simulink model "inverted_pendulum"  (Simulink 6.0)
settings: Solver=ode45  StartTime=0.0  StopTime=10.0  RelTol=1e-3
values from neighbouring files (symbols this model uses):
  B = [0;-1;0;1]    [Invertedpendulum.m]    (also in Untitled.m = [-1;0;2])
  C = eye(4)    [Invertedpendulum.m]    (also in Untitled.m = [0 1 0;0 0 1])
  C1 = C    [Invertedpendulum.m]
  C2 = C    [Invertedpendulum.m]
  C3 = C    [Invertedpendulum.m]
  C4 = C    [Invertedpendulum.m]
  E = [1;1;1;1]    [Invertedpendulum.m]    (also in Untitled.m = [1;0;1])
  F = diag(v)    [Invertedpendulum.m]    (also in Untitled.m = A1-K1'*C)
  F1 = T1*A-k11*C1    [Invertedpendulum.m]
  F3 = T3*A-k31*C3    [Invertedpendulum.m]
  F4 = T4*A-k41*C4    [Invertedpendulum.m]
  H = E*(inv((C*E)'*(C*E)))*(C*E)'    [Invertedpendulum.m]    (also in Untitled.m = E*inv((C*E)'*(C*E))*(C*E)')
  H1 = zeros(4,4)    [Invertedpendulum.m]
  H2 = zeros(4,4)    [Invertedpendulum.m]
  H3 = zeros(4,4)    [Invertedpendulum.m]
  H4 = zeros(4,4)    [Invertedpendulum.m]
  k = k1+k2    [Invertedpendulum.m]
  K1 = k11+k12    [Invertedpendulum.m]    (also in Untitled.m = place(A',C',[-2,-10,-5])')
  K2 = k21+k22    [Invertedpendulum.m]
  K3 = k31+k32    [Invertedpendulum.m]
  K4 = k41+k42    [Invertedpendulum.m]
  T = eye(4)-H*C    [Invertedpendulum.m]    (also in Untitled.m = eye(3)-H*C)
  T1 = eye(4)-H1*C1    [Invertedpendulum.m]
  T2 = eye(4)-H2*C2    [Invertedpendulum.m]
  T3 = eye(4)-H3*C3    [Invertedpendulum.m]
  T4 = eye(4)-H4*C4    [Invertedpendulum.m]
settings Model: LastModifiedBy=fel722

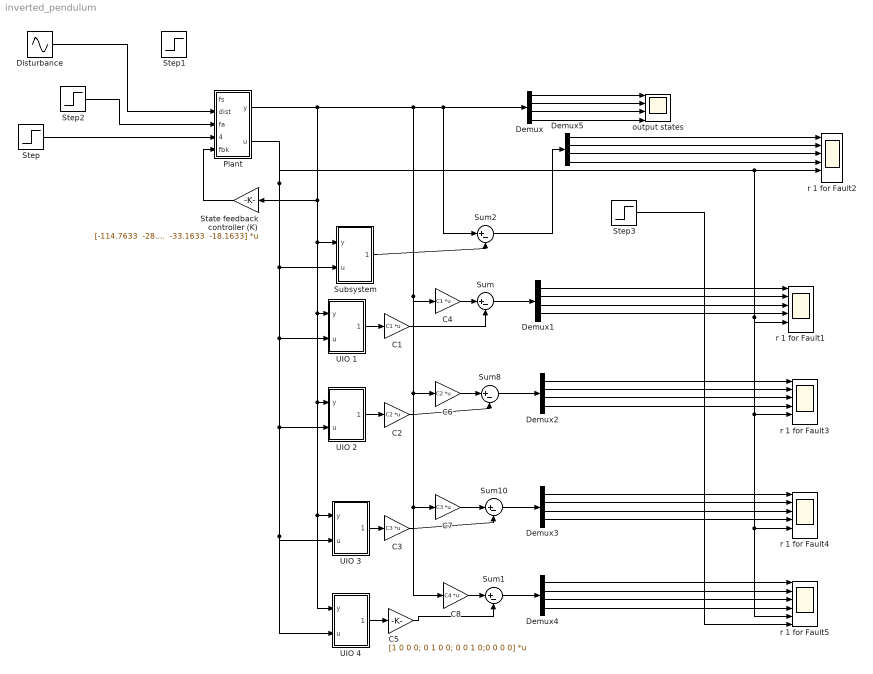
== system inverted_pendulum ==
  C1 : Gain  Gain=C1  Multiplication=Matrix(K*u)
  C2 : Gain  Gain=C2  Multiplication=Matrix(K*u)
  C3 : Gain  Gain=C3  Multiplication=Matrix(K*u)
  C4 : Gain  Gain=C1  Multiplication=Matrix(K*u)
  C5 : Gain  Gain=[1 0 0 0; 0 1 0 0; 0 0 1 0;0 0 0 0]  Multiplication=Matrix(K*u)
  C6 : Gain  Gain=C2  Multiplication=Matrix(K*u)
  C7 : Gain  Gain=C3  Multiplication=Matrix(K*u)
  C8 : Gain  Gain=C4  Multiplication=Matrix(K*u)
  Demux{,1..5} (6 alike) : Demux
  Disturbance : Sin  Amplitude=0.1  Frequency=50  SampleTime=0
  Plant : Subsystem
  State feedback controller (K) : Gain  Orientation=left  Gain="[-114.7633  -28.1633  -33.1633  -18.1633]"  Multiplication=Matrix(K*u)
  Step : Step  Time=0  SampleTime=0
  Step1 : Step  Time=7  SampleTime=0
  Step2 : Step  Time=7  SampleTime=0
  Step3 : Step  Time=7  SampleTime=0
  Subsystem : Subsystem
  Sum{,1..2,8,10} (5 alike) : Sum  Inputs=|+-
  UIO 1 : Subsystem
  UIO 2 : Subsystem
  UIO 3 : Subsystem
  UIO 4 : Subsystem
  output states : Scope  NumInputPorts=4
      settings: TimeRange=10  YMin=-5~-5~-5~-5  YMax=5~5~5~5
  r 1 for Fault{1..5} (5 alike) : Scope  NumInputPorts=6
      r 1 for Fault1 settings: YMin=-5~-5~-5~-5~-5~-5  YMax=5~5~5~5~5~5
      r 1 for Fault2 settings: YMin=-5~-5~-5~-5~-5~-5  YMax=5~5~5~5~5~5  SaveName=ScopeData5
      r 1 for Fault3 settings: YMin=-5~-5~-5~-5~-5~-5  YMax=5~5~5~5~5~5  SaveName=ScopeData3
      r 1 for Fault4 settings: YMin=-5~-5~-5~-5~-5~-5  YMax=5~5~5~5~5~5  SaveName=ScopeData2
      r 1 for Fault5 settings: YMin=-5~-5~-5~-5~-5~-5  YMax=5~5~5~5~5~5  SaveName=ScopeData4
  wires:
  Plant/1(y) -> State feedback controller (K)/1, UIO 1/1(y), UIO 2/1(y), UIO 3/1(y), UIO 4/1(y), Subsystem/1(y), C4/1, C6/1, C7/1, C8/1, Demux/1, Sum2/1
  Demux/1 -> output states/1
  Demux/2 -> output states/2
  Demux/3 -> output states/3
  Demux/4 -> output states/4
  UIO 1/1(xdot) -> C1/1
  C1/1 -> Sum/2
  Sum/1 -> Demux1/1
  UIO 2/1(xdot) -> C2/1
  Sum8/1 -> Demux2/1
  C2/1 -> Sum8/2
  UIO 3/1(xdot) -> C3/1
  Sum10/1 -> Demux3/1
  C3/1 -> Sum10/2
  State feedback controller (K)/1 -> Plant/5(fbk)
  Plant/2(u) -> UIO 1/2(u), UIO 2/2(u), UIO 3/2(u), UIO 4/2(u), Subsystem/2(u), r 1 for Fault2/5, r 1 for Fault1/5, r 1 for Fault3/5, r 1 for Fault4/5, r 1 for Fault5/5
  C4/1 -> Sum/1
  UIO 4/1(xdot) -> C5/1
  C5/1 -> Sum1/2
  Sum1/1 -> Demux4/1
  C6/1 -> Sum8/1
  C7/1 -> Sum10/1
  C8/1 -> Sum1/1
  Subsystem/1(ydot) -> Sum2/2
  Sum2/1 -> Demux5/1
  Demux5/1 -> r 1 for Fault2/1
  Demux5/2 -> r 1 for Fault2/2
  Demux5/3 -> r 1 for Fault2/3
  Demux5/4 -> r 1 for Fault2/4
  Step/1 -> Plant/4(step)
  Step3/1 -> r 1 for Fault5/6
  Demux1/1 -> r 1 for Fault1/1
  Demux1/2 -> r 1 for Fault1/2
  Demux1/3 -> r 1 for Fault1/3
  Demux1/4 -> r 1 for Fault1/4
  Demux2/1 -> r 1 for Fault3/1
  Demux2/2 -> r 1 for Fault3/2
  Demux2/3 -> r 1 for Fault3/3
  Demux2/4 -> r 1 for Fault3/4
  Demux3/1 -> r 1 for Fault4/1
  Demux3/2 -> r 1 for Fault4/2
  Demux3/3 -> r 1 for Fault4/3
  Demux3/4 -> r 1 for Fault4/4
  Demux4/1 -> r 1 for Fault5/1
  Demux4/2 -> r 1 for Fault5/2
  Demux4/3 -> r 1 for Fault5/3
  Demux4/4 -> r 1 for Fault5/4
  Disturbance/1 -> Plant/2(dist)
  Step2/1 -> Plant/3(fa)

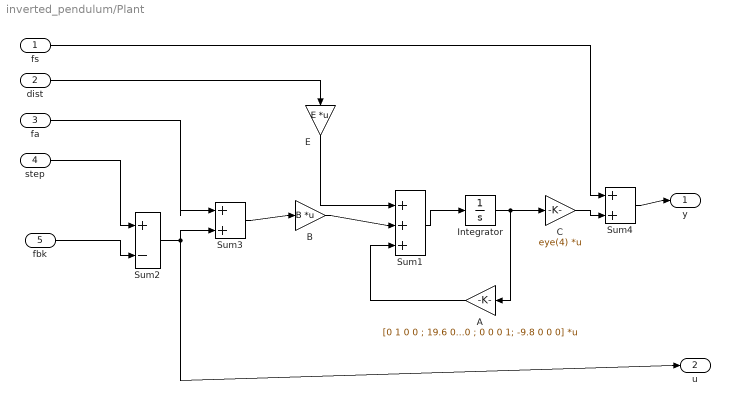
== system inverted_pendulum/Plant ==
  fs : Inport  Port=1  LatchInput=off
  dist : Inport  Port=2  LatchInput=off
  fa : Inport  Port=3  LatchInput=off
  step : Inport  Port=4  LatchInput=off
  fbk : Inport  Port=5  LatchInput=off
  A : Gain  Orientation=left  Gain=[0 1 0 0 ; 19.6 0 0 0 ; 0 0 0 1; -9.8 0 0 0]  Multiplication=Matrix(K*u)
  B : Gain  Gain=B  Multiplication=Matrix(K*u)
  C : Gain  Gain=eye(4)  Multiplication=Matrix(K*u)
  E : Gain  Orientation=down  Gain=E  Multiplication=Matrix(K*u)
  Integrator : Integrator
  Sum1 : Sum  Inputs=|+++
  Sum2 : Sum  Inputs=|+-
  Sum3 : Sum  Inputs=|++
  Sum4 : Sum  Inputs=|++
  y : Outport
  u : Outport  Port=2
  wires:
  Sum1/1 -> Integrator/1
  step/1 -> Sum2/1
  fbk/1 -> Sum2/2
  Integrator/1 -> C/1, A/1
  Sum2/1 -> Sum3/2, u/1
  B/1 -> Sum1/2
  Sum3/1 -> B/1
  C/1 -> Sum4/2
  A/1 -> Sum1/3
  E/1 -> Sum1/1
  Sum4/1 -> y/1
  fa/1 -> Sum3/1
  dist/1 -> E/1
  fs/1 -> Sum4/1

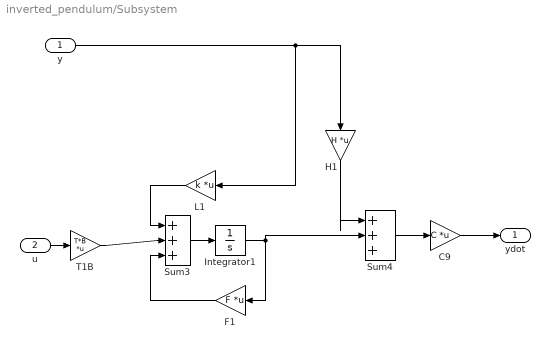
== system inverted_pendulum/Subsystem ==
  y : Inport  Port=1  LatchInput=off
  u : Inport  Port=2  LatchInput=off
  C9 : Gain  Gain=C  Multiplication=Matrix(K*u)
  F1 : Gain  Orientation=left  Gain=F  Multiplication=Matrix(K*u)
  H1 : Gain  Orientation=down  Gain=H  Multiplication=Matrix(K*u)
  Integrator1 : Integrator
  L1 : Gain  Orientation=left  Gain=k  Multiplication=Matrix(K*u)
  Sum3 : Sum  Inputs=|+++
  Sum4 : Sum  Inputs=|+++
  T1B : Gain  Gain=T*B  Multiplication=Matrix(K*u)
  ydot : Outport
  wires:
  Sum3/1 -> Integrator1/1
  Integrator1/1 -> F1/1, Sum4/2
  F1/1 -> Sum3/3
  L1/1 -> Sum3/1
  T1B/1 -> Sum3/2
  H1/1 -> Sum4/1
  Sum4/1 -> C9/1
  y/1 -> L1/1, H1/1
  u/1 -> T1B/1
  C9/1 -> ydot/1

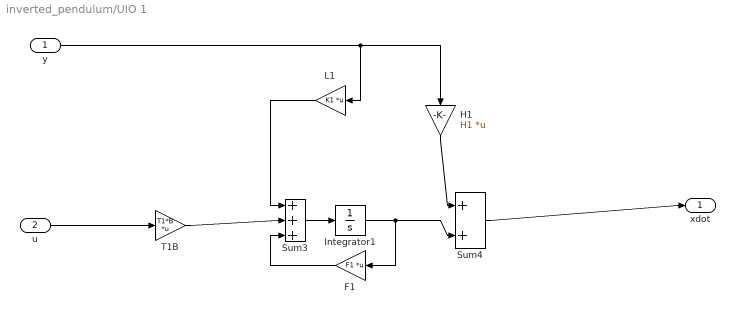
== system inverted_pendulum/UIO 1 ==
  y : Inport  Port=1  LatchInput=off
  u : Inport  Port=2  LatchInput=off
  F1 : Gain  Orientation=left  Gain=F1  Multiplication=Matrix(K*u)
  H1 : Gain  Orientation=down  Gain=H1  Multiplication=Matrix(K*u)
  Integrator1 : Integrator
  L1 : Gain  Orientation=left  Gain=K1  Multiplication=Matrix(K*u)
  Sum3 : Sum  Inputs=|+++
  Sum4 : Sum  Inputs=|++
  T1B : Gain  Gain=T1*B  Multiplication=Matrix(K*u)
  xdot : Outport
  wires:
  Sum3/1 -> Integrator1/1
  Integrator1/1 -> Sum4/2, F1/1
  F1/1 -> Sum3/3
  L1/1 -> Sum3/1
  T1B/1 -> Sum3/2
  H1/1 -> Sum4/1
  u/1 -> T1B/1
  Sum4/1 -> xdot/1
  y/1 -> H1/1, L1/1

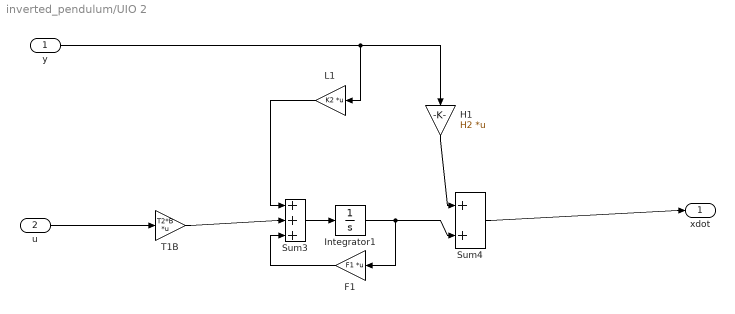
== system inverted_pendulum/UIO 2 ==
  y : Inport  Port=1  LatchInput=off
  u : Inport  Port=2  LatchInput=off
  F1 : Gain  Orientation=left  Gain=F1  Multiplication=Matrix(K*u)
  H1 : Gain  Orientation=down  Gain=H2  Multiplication=Matrix(K*u)
  Integrator1 : Integrator
  L1 : Gain  Orientation=left  Gain=K2  Multiplication=Matrix(K*u)
  Sum3 : Sum  Inputs=|+++
  Sum4 : Sum  Inputs=|++
  T1B : Gain  Gain=T2*B  Multiplication=Matrix(K*u)
  xdot : Outport
  wires:
  Sum3/1 -> Integrator1/1
  Integrator1/1 -> Sum4/2, F1/1
  F1/1 -> Sum3/3
  L1/1 -> Sum3/1
  T1B/1 -> Sum3/2
  H1/1 -> Sum4/1
  u/1 -> T1B/1
  Sum4/1 -> xdot/1
  y/1 -> H1/1, L1/1

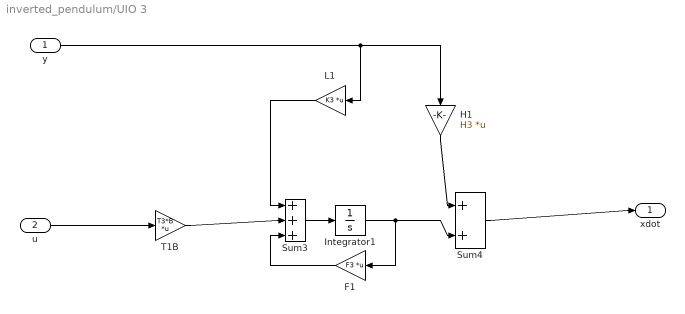
== system inverted_pendulum/UIO 3 ==
  y : Inport  Port=1  LatchInput=off
  u : Inport  Port=2  LatchInput=off
  F1 : Gain  Orientation=left  Gain=F3  Multiplication=Matrix(K*u)
  H1 : Gain  Orientation=down  Gain=H3  Multiplication=Matrix(K*u)
  Integrator1 : Integrator
  L1 : Gain  Orientation=left  Gain=K3  Multiplication=Matrix(K*u)
  Sum3 : Sum  Inputs=|+++
  Sum4 : Sum  Inputs=|++
  T1B : Gain  Gain=T3*B  Multiplication=Matrix(K*u)
  xdot : Outport
  wires:
  Sum3/1 -> Integrator1/1
  Integrator1/1 -> Sum4/2, F1/1
  F1/1 -> Sum3/3
  L1/1 -> Sum3/1
  T1B/1 -> Sum3/2
  H1/1 -> Sum4/1
  u/1 -> T1B/1
  Sum4/1 -> xdot/1
  y/1 -> H1/1, L1/1

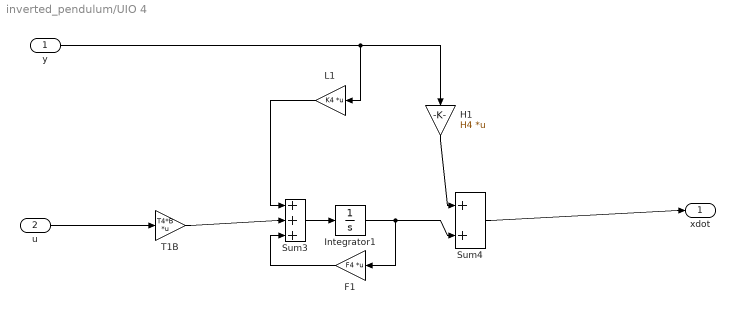
== system inverted_pendulum/UIO 4 ==
  y : Inport  Port=1  LatchInput=off
  u : Inport  Port=2  LatchInput=off
  F1 : Gain  Orientation=left  Gain=F4  Multiplication=Matrix(K*u)
  H1 : Gain  Orientation=down  Gain=H4  Multiplication=Matrix(K*u)
  Integrator1 : Integrator
  L1 : Gain  Orientation=left  Gain=K4  Multiplication=Matrix(K*u)
  Sum3 : Sum  Inputs=|+++
  Sum4 : Sum  Inputs=|++
  T1B : Gain  Gain=T4*B  Multiplication=Matrix(K*u)
  xdot : Outport
  wires:
  Sum3/1 -> Integrator1/1
  Integrator1/1 -> Sum4/2, F1/1
  F1/1 -> Sum3/3
  L1/1 -> Sum3/1
  T1B/1 -> Sum3/2
  H1/1 -> Sum4/1
  u/1 -> T1B/1
  Sum4/1 -> xdot/1
  y/1 -> H1/1, L1/1
